simulink model "Binary_PAM"  (R2016a)
settings: Solver=FixedStepDiscrete  SolverMode=SingleTasking  StartTime=0.0  StopTime=16*(3*7)  RelTol=1e-3
libraries: simulink x1, dspsrcs4 x1, dspsigops x1
settings Model: Creator=coltmt  LastModifiedBy=coltmt
settings DataIOCC: LimitDataPoints=on
settings DebuggingCC: AllowSymbolicDim=off
settings ModelReferenceCC: PropagateSignalLabelsOutOfModel=off
settings GRTTargetCC: GeneratePreprocessorConditionals=Use local settings

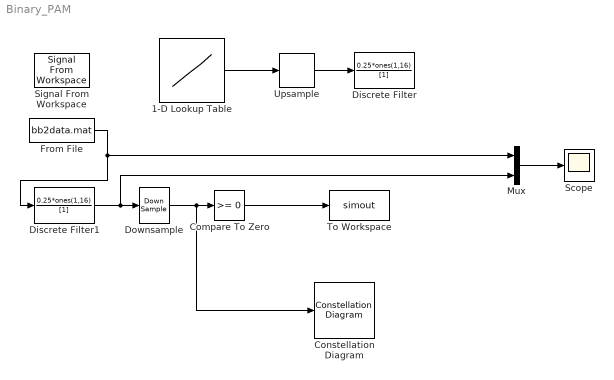
== system Binary_PAM ==
  1-D Lookup Table : Lookup_n-D  NumberOfTableDimensions=1  BreakpointsForDimension1=[0 1]  Table=[-1 1]  InternalRulePriority=Speed  RndMeth=Simplest  InputSameDT=on
  Compare To Zero : simulink/Logic and Bit Operations/Compare To Zero  relop=>=  OutDataTypeStr=boolean
  Constellation Diagram : ConstellationDiagram
  Discrete Filter : DiscreteFilter  Numerator=0.25*ones(1,16)  Denominator=[1]
  Discrete Filter1 : DiscreteFilter  Numerator=0.25*ones(1,16)  Denominator=[1]
  Downsample : DownSample  N=16  phase=15  InputProcessing=Inherited (this choice will be removed - see release notes)  RateOptions=Allow multirate processing
  From File : FromFile  FileName=bb2data.mat  SampleTime=1
  Mux : Mux  Inputs=2
  Scope : Scope
  Signal From Workspace : dspsrcs4/Signal From Workspace  X=[1 0 0 1]  Ts=16  nsamps=1  OutputAfterFinalValue=Setting to zero  ignoreOrWarnInputAndFrameLengths=off  OutputFrames=off
  To Workspace : ToWorkspace  VariableName=simout  SampleTime=-1
      settings: Save2DSignal=2-D array (concatenate along first dimension)
  Upsample : dspsigops/Upsample  N=16  phase=7  InputProcessing=Inherited (this choice will be removed - see release notes)  RateOptions=Allow multirate processing  ic=0  mode=Unused parameter value
  wires:
  1-D Lookup Table/1 -> Upsample/1
  Upsample/1 -> Discrete Filter/1
  Discrete Filter1/1 -> Mux/2, Downsample/1
  Downsample/1 -> Constellation Diagram/1, Compare To Zero/1
  Compare To Zero/1 -> To Workspace/1
  Mux/1 -> Scope/1
  From File/1 -> Mux/1, Discrete Filter1/1
